simulink model "MACARAIG_SIMULINK_NO6"  (R2024a)
settings: Solver=VariableStepAuto  StartTime=0.0  StopTime=10.0  RelTol=1e-3
values from neighbouring files (symbols this model uses):
  g6_den = [d5,d4,d3,d2,d]    [LAB 2 NO. 5 AND NO. 6.m]
  G6_num = [c4,c3,c2,c]    [LAB 2 NO. 5 AND NO. 6.m]

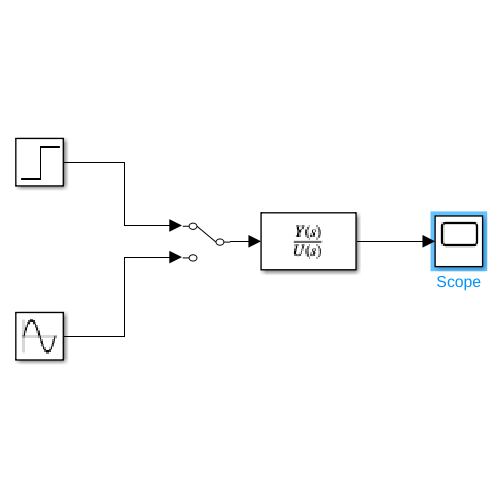
[thumbnail: Simulink's stored preview of the top-level diagram]
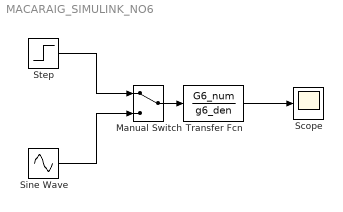
== system MACARAIG_SIMULINK_NO6 ==
  Manual Switch : ManualSwitch
  Scope : Scope
  Sine Wave : Sin  SampleTime=0
  Step : Step  Time=0  SampleTime=0
  Transfer Fcn : TransferFcn  Numerator=G6_num  Denominator=g6_den
  wires:
  Step/1 -> Manual Switch/1
  Sine Wave/1 -> Manual Switch/2
  Manual Switch/1 -> Transfer Fcn/1
  Transfer Fcn/1 -> Scope/1
